simulink model "State_Space_Quarc"  (R2019a)
settings: Solver=FixedStepDiscrete  StartTime=0.0  StopTime=20-.002  FixedStep=0.002  RelTol=1e-3  EnableMultiTasking=on
PostLoadFcn:
  | qc_set_target_type(getConfigSet(bdroot, 'QUARC Default Target Configuration'));
values from neighbouring files (symbols this model uses):
  b = 36.29    [Pendelum_TF2.mat]
  c = 20.51    [Pendelum_TF2.mat]
  dT = 0.002    [Pendulum_SS_Init.m]    (also in Pendulum_SS_Init_Data.mat)
  G = [1, 0]'    [Pendulum_State_Space.m]
  K = place(A,B, [-16, -15])    [Pendulum_State_Space.m]
  Ki = [10 0]    [Pendulum_State_Space.m]
undefined symbols (not defined in the file or in its folder): DiscIntNeverNeededParam, HIL
libraries: quarc_library x4
settings Model: SimulationMode=external  ExtModeTrigDuration=10000  Creator=MLevis  LastModifiedBy=QuarcUser
settings SolverCC: PositivePriorityOrder=on
settings DataIOCC: LimitDataPoints=on  SaveFormat=Array  SignalLoggingSaveFormat=ModelDataLogs  ReturnWorkspaceOutputs=off
settings OptimizationCC: ExpressionDepthLimit=2147483647  InitFltsAndDblsToZero=on  LifeSpan=inf
settings DebuggingCC: SaveWithParameterizedLinksMsg=none  UnderspecifiedInitializationDetection=Classic  MergeDetectMultiDrivingBlocksExec=none  SolverPrmCheckMsg=warning  MultiTaskDSMMsg=warning  MultiTaskCondExecSysMsg=none  FcnCallInpInsideContextMsg=warning  StateNameClashWarn=warning  SFUnexpectedBacktrackingDiag=warning  SFNoUnconditionalDefaultTransitionDiag=warning  SFExecutionAtInitializationDiag=none  ArithmeticOperatorsInVariantConditions=warning
settings HardwareCC: ProdBitPerPointer=32  ProdBitPerSizeT=32  ProdBitPerPtrDiffT=32  ProdLargestAtomicFloat=None  ProdIntDivRoundTo=Undefined  ProdEndianess=Unspecified  ProdWordSize=32  ProdHWDeviceType=32-bit Generic
settings ModelReferenceCC: PropagateSignalLabelsOutOfModel=off
settings SFSimCC: SimUseLocalCustomCode=off
settings RTWCC: SystemTargetFile=quarc_win64.tlc  TemplateMakefile=quarc_default_tmf  Description=QUARC Win64 Target  RTWUseLocalCustomCode=off
settings CodeAppCC: StateflowObjectComments=on
settings STFCustomTargetCC: TargetPreCompLibLocation=C:\PROGRA~3\QUARC\lib\2019a\win64\release  ConcurrentExecutionCompliant=on  GeneratePreprocessorConditionals=Disable all  CPPClassGenCompliant=on  SystemTargetFile=quarc_win64.tlc
settings GRTTargetCC: TargetPreCompLibLocation=C:\PROGRA~3\QUARC\lib\2019a\win64\release  TargetLangStandard=C89/C90 (ANSI)  ParMdlRefBuildCompliant=off  CompOptLevelCompliant=off  GeneratePreprocessorConditionals=Disable all  CombineOutputUpdateFcns=off  MatFileLogging=off  GRTInterface=on  UseToolchainInfoCompliant=off  ExtMode=on  ExtModeMexFile=quarc_comm
settings ConfigComp: CovMetricSettings=dw  CovHtmlReporting=on  CovSaveCumulativeToWorkspaceVar=on  CovSaveSingleToWorkspaceVar=on  CovExternalEMLEnable=off

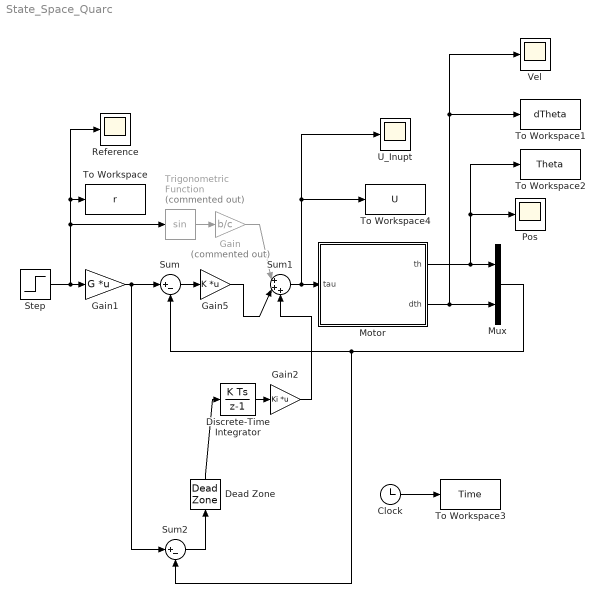
== system State_Space_Quarc ==
  Clock : Clock
  Dead Zone : DeadZone  LowerValue=-0.05  UpperValue=0.05  SaturateOnIntegerOverflow=on
  Discrete-Time Integrator : DiscreteIntegrator  SampleTime=dT  ICPrevOutput=DiscIntNeverNeededParam  ICPrevScaledInput=DiscIntNeverNeededParam
  Gain : Gain  Commented=on  Gain=b/c
  Gain1 : Gain  Gain=G  Multiplication=Matrix(K*u)
  Gain2 : Gain  Gain=Ki  Multiplication=Matrix(K*u)
  Gain5 : Gain  Gain=K  Multiplication=Matrix(K*u)
  Motor : Subsystem
  Mux : Mux  Inputs=2
  Pos : Scope
  Reference : Scope
  Step : Step  SampleTime=dT
  Sum : Sum  Inputs=|+-
  Sum1 : Sum  Inputs=|+++
  Sum2 : Sum  Inputs=|+-
  To Workspace : ToWorkspace  VariableName=r  SampleTime=-1
  To Workspace1 : ToWorkspace  VariableName=dTheta  SampleTime=-1
  To Workspace2 : ToWorkspace  VariableName=Theta  SampleTime=-1
  To Workspace3 : ToWorkspace  VariableName=Time  SampleTime=-1
  To Workspace4 : ToWorkspace  VariableName=U  SampleTime=-1
  Trigonometric Function : Trigonometry  Commented=on
  U_Inupt : Scope
  "Vel " : Scope
  wires:
  Clock/1 -> To Workspace3/1
  Step/1 -> Gain1/1, Trigonometric Function/1, Reference/1, To Workspace/1
  Gain1/1 -> Sum2/1, Sum/1
  Sum/1 -> Gain5/1
  Motor/2(dth) -> Mux/2, "Vel "/1, To Workspace1/1
  Gain5/1 -> Sum1/2
  Mux/1 -> Sum2/2, Sum/2
  Motor/1(th) -> Mux/1, Pos/1, To Workspace2/1
  Sum1/1 -> U_Inupt/1, To Workspace4/1, Motor/1(tau)
  Trigonometric Function/1 -> Gain/1
  Gain/1 -> Sum1/1
  Gain2/1 -> Sum1/3
  Sum2/1 -> Dead Zone/1
  Discrete-Time Integrator/1 -> Gain2/1
  Dead Zone/1 -> Discrete-Time Integrator/1

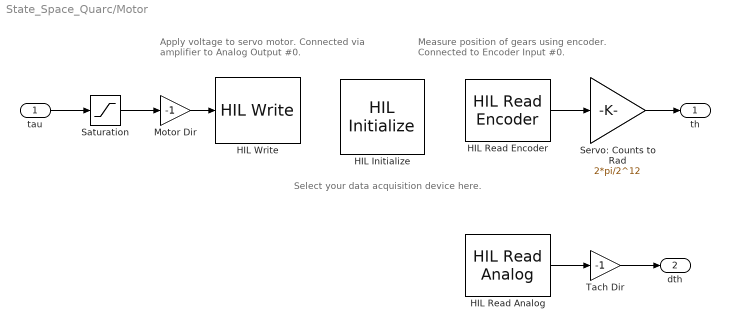
== system State_Space_Quarc/Motor ==
  note: Apply voltage to servo motor.
      | Connected via amplifier to Analog Output #0.
  note: Measure position of gears using encoder.
      | Connected to Encoder Input #0.
  note: Select your data acquisition device here.
  tau : Inport
  HIL Initialize : quarc_library/Data Acquisition/Generic/Configuration/HIL Initialize  object_name=HIL-1  board_type=q2_usb  board_number=0  board_options=d0=digital;d1=digital;led=auto;update_rate=normal;decimation=1  exclusive=off  active=off  hardware_clocks=[0]  clock_modes=[]  initial_clock_frequencies=[]  set_clock_params_at_start=off  set_clock_params_at_switch_in=off  set_clock_frequencies_at_start=off  set_clock_frequencies_at_switch_in=off  analog_input_channels=[0:1]  analog_input_configurations=[]  analog_input_maximums=10  analog_input_minimums=-10  set_analog_input_params_at_start=on  set_analog_input_params_at_switch_in=off  analog_output_channels=[0:1]  analog_output_maximums=10  analog_output_minimums=-10  initial_analog_outputs=[0]  final_analog_outputs=[0]  watchdog_analog_outputs=0  set_analog_output_params_at_start=on  set_analog_output_params_at_switch_in=off  set_analog_outputs_at_start=on  set_analog_outputs_at_switch_in=off  set_analog_outputs_at_terminate=on  set_analog_outputs_at_switch_out=off  set_analog_outputs_on_watchdog=off  digital_input_channels=[]  digital_output_channels=[]  digital_output_configuration=[]  initial_digital_outputs=[1]  final_digital_outputs=[1]  watchdog_digital_outputs=[1]  set_digital_output_params_at_start=off  set_digital_output_params_at_switch_in=off  set_digital_outputs_at_start=on  set_digital_outputs_at_switch_in=off  set_digital_outputs_at_terminate=on  set_digital_outputs_at_switch_out=off  set_digital_outputs_on_watchdog=off  encoder_channels=[0:1]  quadrature=[4]  encoder_filter_frequency=[]  initial_encoder_counts=[0]  set_encoder_params_at_start=on  set_encoder_params_at_switch_in=off  set_encoder_counts_at_start=on  set_encoder_counts_at_switch_in=off  pwm_channels=[]  pwm_modes=[0]  pwm_frequency=1/0.020  pwm_configuration=[]  pwm_alignment=[]  pwm_polarity=[]  pwm_leading_deadband=[]  pwm_trailing_deadband=[]  initial_pwm_outputs=[0]  final_pwm_outputs=[0]  watchdog_pwm_outputs=[0]  set_pwm_params_at_start=on  set_pwm_params_at_switch_in=off  set_pwm_outputs_at_start=on  set_pwm_outputs_at_switch_in=off  set_pwm_outputs_at_terminate=on  set_pwm_outputs_at_switch_out=off  set_pwm_outputs_on_watchdog=off  other_output_channels=[]  initial_other_outputs=[]  final_other_outputs=[]  watchdog_other_outputs=[]  set_other_outputs_at_start=off  set_other_outputs_at_switch_in=off  set_other_outputs_at_terminate=off  set_other_outputs_at_switch_out=off  set_other_outputs_on_watchdog=off
  HIL Read Analog : quarc_library/Data Acquisition/Generic/Immediate I//O/HIL Read Analog  object_name=HIL-1  channels=[0]  sample_time=qc_get_step_size  active=on  vector_output=off
  HIL Read Encoder : quarc_library/Data Acquisition/Generic/Immediate I//O/HIL Read Encoder  object_name=HIL-1  channels=0  sample_time=qc_get_step_size  active=on  vector_output=off  data_type_mode=Inherit via back propagation  data_type=double
  HIL Write : quarc_library/Data Acquisition/Generic/Immediate I//O/HIL Write  Tag=unassigned  object_name=HIL-1  analog_channels=0  pwm_channels=[]  digital_channels=[]  other_channels=[]  sample_time=-1  active=off  vector_input=off
  "Motor Dir " : Gain  Gain=-1
  Saturation : Saturate  UpperLimit=10  LowerLimit=-10
  Servo: Counts to Rad : Gain  Gain=2*pi/2^12
  Tach Dir : Gain  Gain=-1
  th : Outport
  dth : Outport  Port=2
  wires:
  Saturation/1 -> "Motor Dir "/1
  HIL Read Encoder/1 -> Servo: Counts to Rad/1
  "Motor Dir "/1 -> HIL Write/1
  tau/1 -> Saturation/1
  Servo: Counts to Rad/1 -> th/1
  HIL Read Analog/1 -> Tach Dir/1
  Tach Dir/1 -> dth/1
